simulink model "lab2simulink"  (R2019b)
settings: Solver=ode45  StartTime=0.0  StopTime=0.2  RelTol=1e-3
settings Model: Creator=wesle  LastModifiedBy=wesle
settings OptimizationCC: BooleanDataType=off

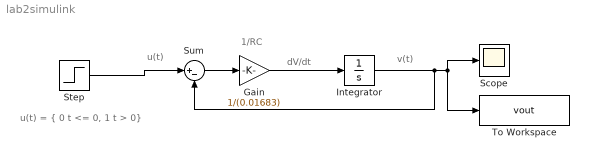
== system lab2simulink ==
  note: u(t) = { 0 t <= 0, 1 t > 0}
  note: v(t)
  note: dV/dt
  note: 1/RC
  note: u(t)
  Gain : Gain  Gain=1/(0.01683)
  Integrator : Integrator
  Scope : Scope
  Step : Step  Time=0  SampleTime=0
  Sum : Sum  Inputs=|+-
  To Workspace : ToWorkspace  VariableName=vout  SampleTime=-1
  wires:
  Sum/1 -> Gain/1
  Integrator/1 -> To Workspace/1, Scope/1, Sum/2
  Gain/1 -> Integrator/1
  Step/1 -> Sum/1
